simulink subsystem "fan"  (R2020b)
settings: Solver=VariableStepAuto  StartTime=0.0  StopTime=10.0  RelTol=1e-3
undefined symbols (not defined in the file): CFM2CMS, rho, tauFan, V2CFM
settings Model: Creator=jclinton  LastModifiedBy=jclinton
settings DebuggingCC: SFMachineParentedDataDiag=error

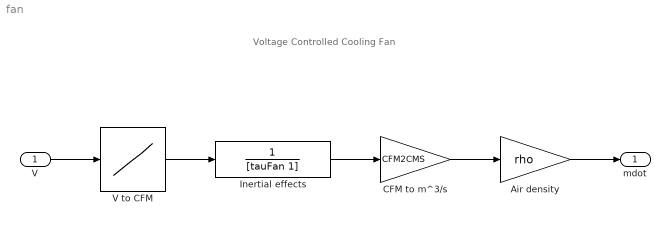
== system fan ==
  note: Voltage Controlled Cooling Fan
  V : Inport  Unit=V
  Air density : Gain  Gain=rho
  CFM to m^3/s : Gain  Gain=CFM2CMS
  Inertial effects : TransferFcn  Denominator=[tauFan 1]
  V to CFM : Lookup_n-D  NumberOfTableDimensions=1  BreakpointsForDimension1=V2CFM(:,1)  Table=V2CFM(:,2)  ExtrapMethod=Clip  InternalRulePriority=Speed  RndMeth=Simplest  InputSameDT=on
  mdot : Outport  Unit=kg/sec
  wires:
  V/1 -> V to CFM/1
  V to CFM/1 -> Inertial effects/1
  Inertial effects/1 -> CFM to m^3/s/1
  CFM to m^3/s/1 -> Air density/1
  Air density/1 -> mdot/1
